simulink model "model"  (R2013b)
settings: Solver=ode45  StartTime=0.0  StopTime=10  FixedStep=0.001  RelTol=1e-3
values from neighbouring files (symbols this model uses):
  alphaF_offset = -3/360*2*pi    (= -0.0523598775598)    [parameters.m]
  alphaR_offset = -3/360*2*pi    (= -0.0523598775598)    [parameters.m]
  g = 9.81    [parameters.m]
  l_p = sqrt(0.115^2 + h_CG^2)    [parameters.m]
  l_w = 0.30    (= 0.3)    [parameters.m]    (also in testing.m = 0.4)
  m_car = 0.7    [dynamics_constants.m]    (also in parameters.m = 1.2)
  v_R = 1 + 0.2*randn    [analyze_parameter_impcact.m]    (also in parameters.m = 1)
  w_w = 250    [parameters.m]    (also in simulation.m)
  w_z = 1.5    [parameters.m]    (also in simulation.m)
undefined symbols (not defined in the file or in its folder): sigbuilder_block
libraries: simulink x1
settings Model: Creator=daniel  LastModifiedBy=daniel
settings ModelReferenceCC: ModelReferenceNumInstancesAllowed=Single

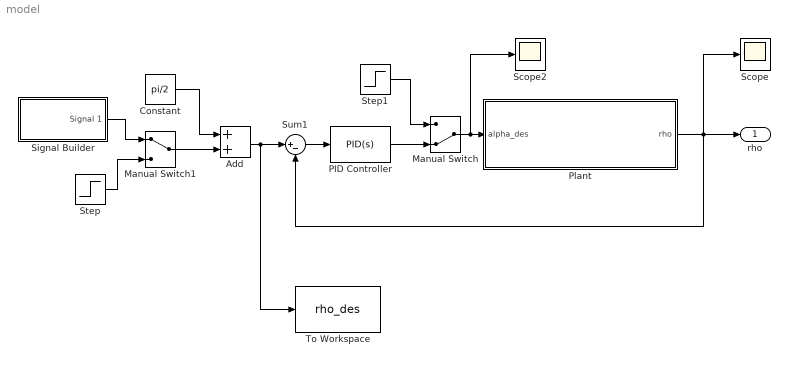
== system model ==
  Add : Sum
  Constant : Constant  Value=pi/2
  Manual Switch : ManualSwitch  CurrentSetting=0
  Manual Switch1 : ManualSwitch
  PID Controller : simulink/Continuous/PID Controller  Controller=PID  TimeDomain=Continuous-time  SampleTime=1  IntegratorMethod=Forward Euler  FilterMethod=Forward Euler  Form=Parallel  P=-12.1789515819894  I=-8.69463644131183  D=-3.79043760517622  N=13984.9608527094  InitialConditionSource=internal  InitialConditionForIntegrator=0  InitialConditionForFilter=0  ExternalReset=none  LimitOutput=on  UpperSaturationLimit=0.25  LowerSaturationLimit=-0.25  LinearizeAsGain=on  AntiWindupMode=clamping  Kb=1  TrackingMode=off  Kt=1  PParamMin=[]  PParamMax=[]  IParamMin=[]  IParamMax=[]  DParamMin=[]  DParamMax=[]  NParamMin=[]  NParamMax=[]  KbParamMin=[]  KbParamMax=[]  KtParamMin=[]  KtParamMax=[]  POutMin=[]  POutMax=[]  IOutMin=[]  IOutMax=[]  DOutMin=[]  DOutMax=[]  NOutMin=[]  NOutMax=[]  KbOutMin=[]  KbOutMax=[]  KtOutMin=[]  KtOutMax=[]  IntegratorOutMin=[]  IntegratorOutMax=[]  FilterOutMin=[]  FilterOutMax=[]  SumOutMin=[]  SumOutMax=[]  SumI1OutMin=[]  SumI1OutMax=[]  SumI2OutMin=[]  SumI2OutMax=[]  SumI3OutMin=[]  SumI3OutMax=[]  SumDOutMin=[]  SumDOutMax=[]  SaturationOutMin=[]  SaturationOutMax=[]  IntegratorContinuousStateAttributes=''  IntegratorStateMustResolveToSignalObject=off  IntegratorRTWStateStorageClass=Auto  FilterContinuousStateAttributes=''  FilterStateMustResolveToSignalObject=off  FilterRTWStateStorageClass=Auto
  Plant : Subsystem
  Scope : Scope
  Scope2 : Scope
      settings: SaveName=ScopeData8
  Signal Builder : Subsystem  Tag=STV Subsys  LoadFcn=sigbuilder_block('load');  StartFcn=sigbuilder_block('start');  StopFcn=sigbuilder_block('stop');  ClipboardFcn=sigbuilder_block('clipboard');  mask(Sigbuilder block){}
      mask help: Simulink:masks:SigbuilderBlock_MD
      mask init:
      | if ~strcmp(get_param(bdroot(gcbh),'SimulationStatus'),'stopped') tuvar = sigbuilder_block('maskInit'); end
      settings: CopyFcn=sigbuilder_block('copy');  DeleteFcn=sigbuilder_block('delete');  ModelCloseFcn=sigbuilder_block('modelClose');  PreSaveFcn=sigbuilder_block('preSave');  PauseFcn=sigbuilder_block('pause');  ContinueFcn=sigbuilder_block('continue');  NameChangeFcn=sigbuilder_block('namechange');  OpenFcn=sigbuilder_block('open',[151.5 69 550.5 395.25 ]);  CloseFcn=sigbuilder_block('close');
      mask Display: plot(0, 0, 100, 100,[2, 2, 32, 32, 2], [68, 8, 8, 68, 68],[32, 2], [38, 38], [32, 19, 2],[53, 60, 44], [32, 17, 17, 2],[16, 16, 31, 31]);txt = getActiveGroup(gcbh);text(2, 100, txt,'verticalAlignment', 'top');
  Step : Step  After=0.3  SampleTime=0.01
  Step1 : Step  Time=0  After=0.3  SampleTime=0.01
  Sum1 : Sum  Inputs=|+-
  To Workspace : ToWorkspace  VariableName=rho_des  SampleTime=-1  SaveFormat=Timeseries
  rho : Outport
  wires:
  Plant/1(rho) -> Sum1/2, rho/1, Scope/1
  Sum1/1 -> PID Controller/1
  PID Controller/1 -> Manual Switch/2
  Manual Switch/1 -> Scope2/1, Plant/1(alpha_des)
  Step1/1 -> Manual Switch/1
  Step/1 -> Manual Switch1/2
  Signal Builder/1(Signal 1) -> Manual Switch1/1
  Add/1 -> To Workspace/1, Sum1/1
  Manual Switch1/1 -> Add/2
  Constant/1 -> Add/1

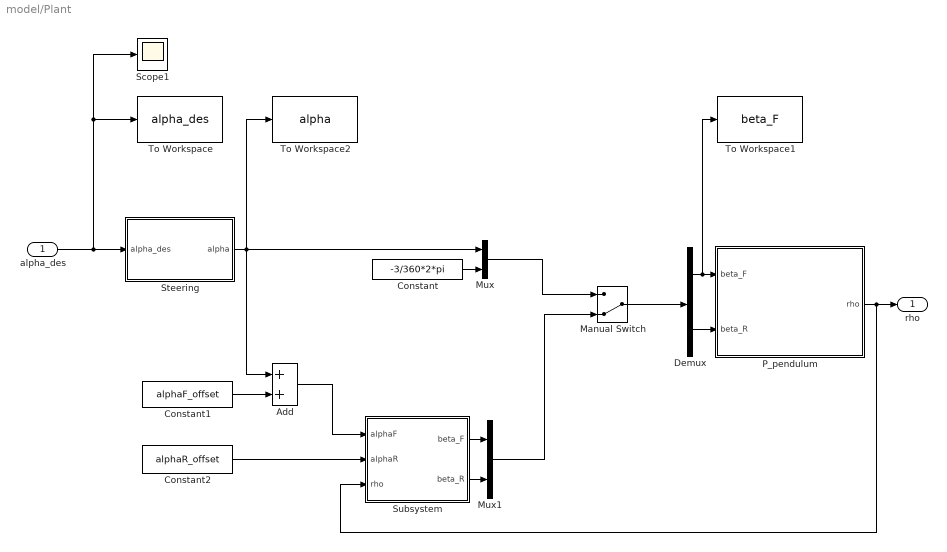
== system model/Plant ==
  alpha_des : Inport
  Add : Sum
  Constant : Constant  Value=-3/360*2*pi
  Constant1 : Constant  Value=alphaF_offset
  Constant2 : Constant  Value=alphaR_offset
  Demux : Demux  Outputs=2
  Manual Switch : ManualSwitch  CurrentSetting=0
  Mux : Mux  Inputs=2
  Mux1 : Mux  Inputs=2
  P_pendulum : Subsystem
  Scope1 : Scope
      settings: SaveName=ScopeData5
  Steering : Subsystem
  Subsystem : Subsystem
  To Workspace : ToWorkspace  VariableName=alpha_des  SampleTime=-1  SaveFormat=Timeseries
  To Workspace1 : ToWorkspace  VariableName=beta_F  SampleTime=-1  SaveFormat=Timeseries
  To Workspace2 : ToWorkspace  VariableName=alpha  SampleTime=-1  SaveFormat=Timeseries
  rho : Outport
  wires:
  Constant/1 -> Mux/2
  P_pendulum/1(rho) -> Subsystem/3(rho), rho/1
  Steering/1(alpha) -> Add/1, To Workspace2/1, Mux/1
  alpha_des/1 -> Scope1/1, To Workspace/1, Steering/1(alpha_des)
  Subsystem/1(beta_F) -> Mux1/1
  Subsystem/2(beta_R) -> Mux1/2
  Demux/1 -> To Workspace1/1, P_pendulum/1(beta_F)
  Demux/2 -> P_pendulum/2(beta_R)
  Manual Switch/1 -> Demux/1
  Mux/1 -> Manual Switch/1
  Mux1/1 -> Manual Switch/2
  Constant1/1 -> Add/2
  Constant2/1 -> Subsystem/2(alphaR)
  Add/1 -> Subsystem/1(alphaF)

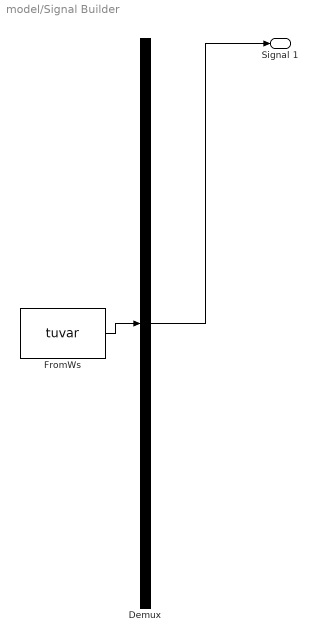
== system model/Signal Builder ==
  Demux : Demux  Tag=STV Demux  Outputs=1
  FromWs : FromWorkspace  Tag=STV FromWs  VariableName=tuvar  SampleTime=0.01
      SigBuilderData=|
      | common.afterFinalStr = 'Extrapolate'
      | common.sampleTime = '0.01'
      | dataSet.timeRange = [0 10]
      | dataSet.name = 'Group 1'
      | sbobj.Groups.Name = 'Group 1'
      | sbobj.Groups.Signals.Name = 'Signal 1'
      | sbobj.Groups.Signals.XData = [0 2.68 2.68 6 6 10]
      | sbobj.Groups.Signals.YData = [-0.051 -0.051 0.066 0.066 0 0]
  Signal 1 : Outport  Tag=STV Outport
  wires:
  Demux/1 -> Signal 1/1
  FromWs/1 -> Demux/1

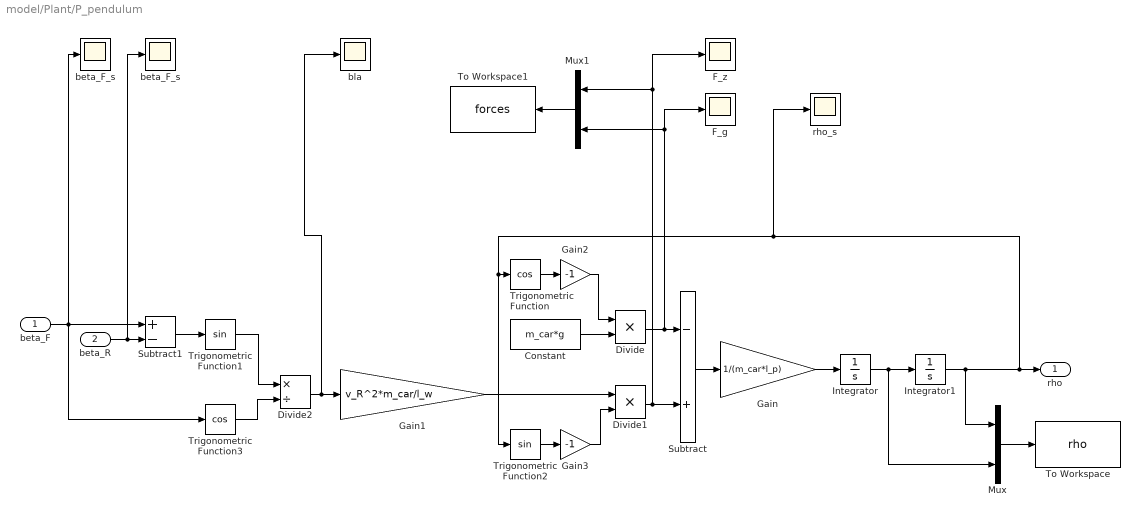
== system model/Plant/P_pendulum ==
  beta_F : Inport
  beta_R : Inport  Port=2
  Constant : Constant  Value=m_car*g
  Divide : Product  Inputs=**
  Divide1 : Product  Inputs=**
  Divide2 : Product  Inputs=*/
  F_g : Scope
      settings: SaveName=ScopeData2
  F_z : Scope
  Gain : Gain  Gain=1/(m_car*l_p)
  Gain1 : Gain  Gain=v_R^2*m_car/l_w
  Gain2 : Gain  Gain=-1
  Gain3 : Gain  Gain=-1
  Integrator : Integrator  ContinuousStateAttributes='rho_dot'
  Integrator1 : Integrator  InitialCondition=pi/2+0.01  ContinuousStateAttributes='rho'
  Mux : Mux  Inputs=2
  Mux1 : Mux  Inputs=2
  Subtract : Sum  Inputs=-+
  Subtract1 : Sum  Inputs=+-
  To Workspace : ToWorkspace  VariableName=rho  SampleTime=-1  SaveFormat=Timeseries
  To Workspace1 : ToWorkspace  VariableName=forces  SampleTime=-1  SaveFormat=Timeseries
  Trigonometric Function : Trigonometry  Operator=cos
  Trigonometric Function1 : Trigonometry
  Trigonometric Function2 : Trigonometry
  Trigonometric Function3 : Trigonometry  Operator=cos
  beta_F_s : Scope
      settings: SaveName=ScopeData7
  "beta_F_s " : Scope
      settings: SaveName=ScopeData9
  bla : Scope
      settings: SaveName=ScopeData10
  rho_s : Scope
      settings: SaveName=ScopeData3
  rho : Outport
  wires:
  Integrator/1 -> Mux/2, Integrator1/1
  Divide1/1 -> F_z/1, Mux1/1, Subtract/2
  Divide/1 -> F_g/1, Mux1/2, Subtract/1
  beta_F/1 -> beta_F_s/1, Trigonometric Function3/1, Subtract1/1
  beta_R/1 -> "beta_F_s "/1, Subtract1/2
  Trigonometric Function1/1 -> Divide2/1
  Trigonometric Function/1 -> Gain2/1
  Divide2/1 -> bla/1, Gain1/1
  Gain/1 -> Integrator/1
  Subtract/1 -> Gain/1
  Subtract1/1 -> Trigonometric Function1/1
  Trigonometric Function2/1 -> Gain3/1
  Mux/1 -> To Workspace/1
  Gain1/1 -> Divide1/1
  Constant/1 -> Divide/2
  Mux1/1 -> To Workspace1/1
  Trigonometric Function3/1 -> Divide2/2
  Integrator1/1 -> rho_s/1, Trigonometric Function2/1, Trigonometric Function/1, rho/1, Mux/1
  Gain2/1 -> Divide/1
  Gain3/1 -> Divide1/2

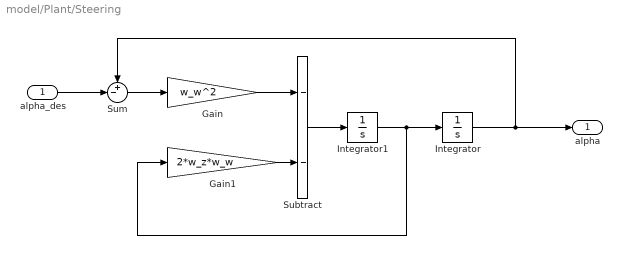
== system model/Plant/Steering ==
  alpha_des : Inport
  Gain : Gain  Gain=w_w^2
  Gain1 : Gain  Gain=2*w_z*w_w
  Integrator : Integrator
  Integrator1 : Integrator
  Subtract : Sum  Inputs=--
  Sum : Sum  Inputs=+-|
  alpha : Outport
  wires:
  Integrator/1 -> alpha/1, Sum/1
  Subtract/1 -> Integrator1/1
  Sum/1 -> Gain/1
  Integrator1/1 -> Gain1/1, Integrator/1
  Gain/1 -> Subtract/1
  Gain1/1 -> Subtract/2
  alpha_des/1 -> Sum/2

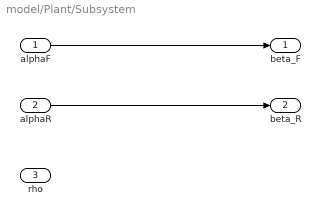
== system model/Plant/Subsystem ==
  alphaF : Inport
  alphaR : Inport  Port=2
  rho : Inport  Port=3
  beta_F : Outport
  beta_R : Outport  Port=2
  wires:
  alphaR/1 -> beta_R/1
  alphaF/1 -> beta_F/1
